simulink model "gm_UZ_EnDat_be4_segregation"  (R2023b)
settings: Solver=FixedStepAuto  StartTime=0  StopTime=0.000505  RelTol=1e-3
model workspace (MAT data in the model file):
  Select = 0
libraries: hdlsllib x74, simulink x21, hdlmdlgenlib x4, simulink_extras x1
(part 1 of 5)
settings Model: SimulationMode=accelerator  Creator=ELSYS_PC  LastModifiedBy=ELSYS_PC
settings SolverCC: AlgebraicLoopSolver=TrustRegion
settings DataIOCC: LimitDataPoints=on  SaveOutput=off  SaveTime=off
settings OptimizationCC: BlockReduction=off  ConditionallyExecuteInputs=off  DefaultParameterBehavior=Inlined  InheritOutputTypeSmallerThanSingle=on  LifeSpan=inf
settings DebuggingCC: AlgebraicLoopMsg=error  ArtificialAlgebraicLoopMsg=none  InheritedTsInSrcMsg=none  SingleTaskRateTransMsg=error  UnconnectedInputMsg=warning  UnconnectedOutputMsg=warning  UnconnectedLineMsg=warning  AllowSymbolicDim=off  StrictBusMsg=ErrorOnBusTreatedAsVector  SFUnexpectedBacktrackingDiag=warning  SFNoUnconditionalDefaultTransitionDiag=warning  SFExecutionAtInitializationDiag=none  ArithmeticOperatorsInVariantConditions=warning
settings HardwareCC: ProdBitPerPointer=32  ProdBitPerSizeT=32  ProdBitPerPtrDiffT=32  ProdLargestAtomicFloat=None  ProdIntDivRoundTo=Undefined  ProdEndianess=Unspecified  ProdWordSize=32  ProdHWDeviceType=ASIC/FPGA->ASIC/FPGA  ProdEqTarget=off
settings ModelReferenceCC: EnableRefExpFcnMdlSchedulingChecks=on
settings SFSimCC: SimUseLocalCustomCode=off  CustomCodeUndefinedFunction=UseInterfaceOnly
settings RTWCC: RTWUseLocalCustomCode=off
settings CodeAppCC: StateflowObjectComments=on
settings GRTTargetCC: TargetLangStandard=C89/C90 (ANSI)  RTWCAPISignals=on  RTWCAPIParams=on
settings ConfigComp: CovScope=ReferencedModels  CovMetricSettings=dw  CovSaveCumulativeToWorkspaceVar=on  CovSaveSingleToWorkspaceVar=on  CovExternalEMLEnable=off  CovSFcnEnable=off  DVTestSuiteOptimization=Auto  DVDetectOutOfBounds=on  DVModelReferenceHarness=on  DVHarnessSource=Signal Editor  DVRebuildModelRepresentation=IfChangeIsDetected

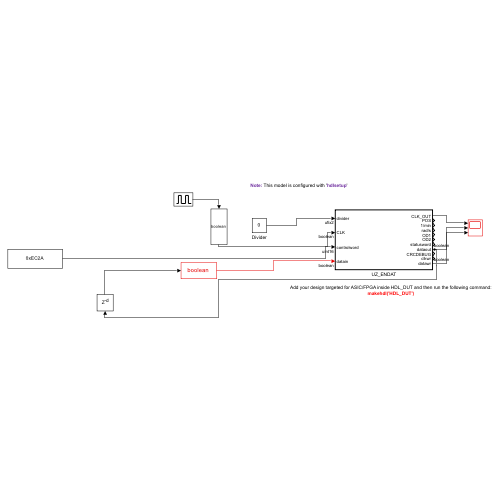
[thumbnail: Simulink's stored preview of the top-level diagram]
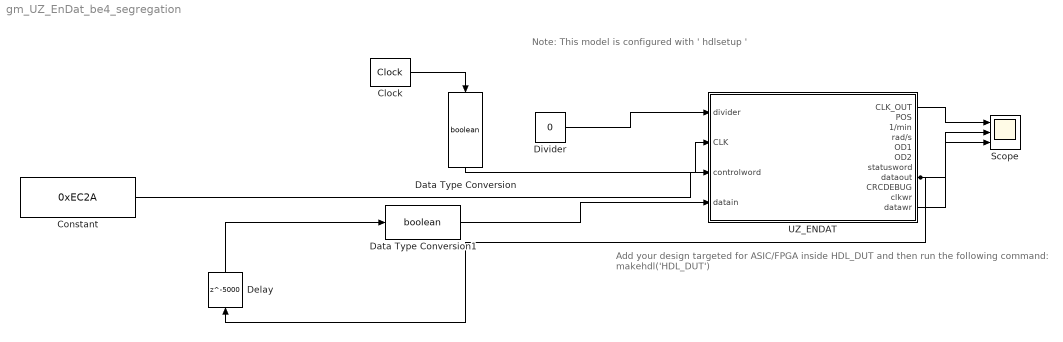
== system gm_UZ_EnDat_be4_segregation ==
  note: Add your design targeted for ASIC/FPGA inside HDL_DUT and then run the following command:
      | makehdl('HDL_DUT')
  note: Note: This model is configured with ' hdlsetup '
  Clock : simulink_extras/Flip Flops/Clock  period=2E-8
  Constant : Constant  Value=0xEC2A  OutDataTypeStr=uint16  SampleTime=-1
  Data Type Conversion : DataTypeConversion  OutDataTypeStr=boolean  SaturateOnIntegerOverflow=off  RndMeth=Floor
  Data Type Conversion1 : DataTypeConversion  OutDataTypeStr=boolean  SaturateOnIntegerOverflow=off  RndMeth=Floor
  Delay : Delay  DelayLength=5000
  Divider : Constant  Value=0  OutMin=0  OutMax=3  OutDataTypeStr=fixdt(0,2,0)  SampleTime=-1
  Scope : Scope  NumInputPorts=3
  UZ_ENDAT : Subsystem  TreatAsAtomicUnit=on
  wires:
  UZ_ENDAT/11(datawr) -> Scope/3
  UZ_ENDAT/1(CLK_OUT) -> Scope/1
  Delay/1 -> Data Type Conversion1/1
  UZ_ENDAT/8(dataout) -> Delay/1, Scope/2
  Data Type Conversion1/1 -> UZ_ENDAT/4(datain)
  Clock/1 -> Data Type Conversion/1
  Divider/1 -> UZ_ENDAT/1(divider)
  Data Type Conversion/1 -> UZ_ENDAT/2(CLK)
  Constant/1 -> UZ_ENDAT/3(controlword)

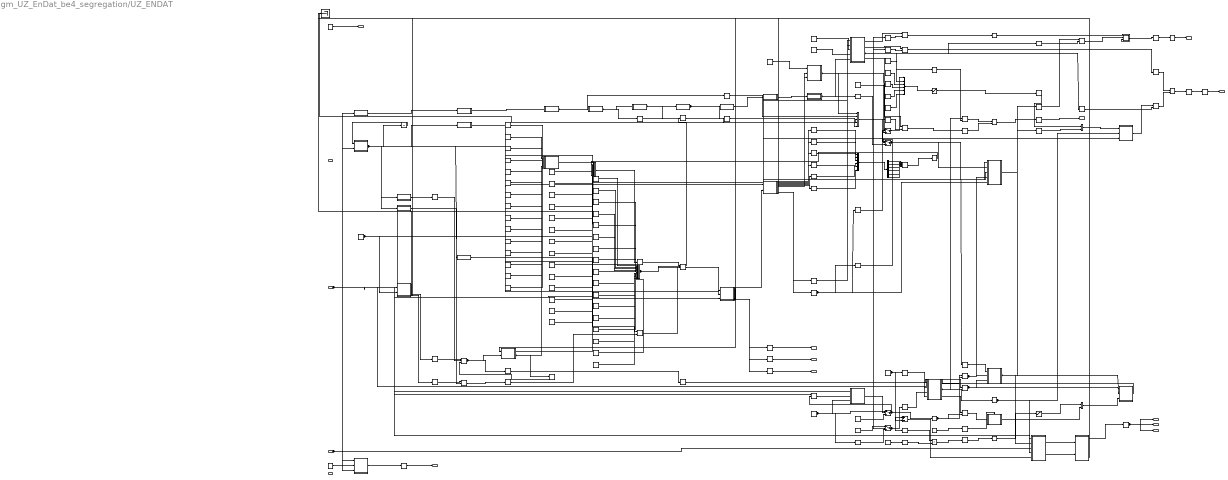
== system gm_UZ_EnDat_be4_segregation/UZ_ENDAT ==
  note: 0=12.5;1=6,25;2=3,125;3=1,5625
  divider : Inport  OutDataTypeStr=fixdt(0, 2, 0)  PortDimensions=1  SampleTime=1e-08
  CLK : Inport  Port=2  OutDataTypeStr=boolean  PortDimensions=1  SampleTime=1e-08
  controlword : Inport  Port=3  OutDataTypeStr=uint16  PortDimensions=1  SampleTime=1e-08
  datain : Inport  Port=4  OutDataTypeStr=boolean  PortDimensions=1  SampleTime=1e-08
  16BIT_SPLITTER : Subsystem
  16BIT_SPLITTER_term{2..14} (13 alike) : Terminator
  16bitgather : Subsystem
  2CLKDELAY : simulink/Discrete/Tapped Delay  vinit=0  samptime=-1  NumDelays=double(1024)  DelayOrder=Newest  includeCurrent=on
  5timestorage : Subsystem
  5timestorage_term{1..4} (4 alike) : Terminator
  CLKCNTER_ACT : Subsystem
  CLKCNTER_RAMPUP : Subsystem
  CLKDIV1 : Subsystem
  CLKDIV2 : Subsystem
  CLKDIV3 : Subsystem
  CLKDIV4 : Subsystem
  CLKDIV5 : Subsystem
  CLKDIV6 : Subsystem
  CLKDIV7 : Subsystem
  CLKDIV8 : Subsystem
  CLKDIV9 : Subsystem
  CONTROLWORDRAW : Subsystem
  CONTROLWORDRAW_term{0..12,14} (14 alike) : Terminator
  CONTROLWORDSTORED : Subsystem
  CONTROLWORDSTORED_term{7..13,15} (8 alike) : Terminator
  CRC_Check : Subsystem
  Compare To Constant : Subsystem  mask(Compare To Constant){relop===, const=double(1), OutDataTypeStr=boolean, ZeroCross=on}
      mask prompts: relop "Simulink:masks:Operator_MP"; const "Simulink:masks:ConstantValue_MP"; OutDataTypeStr "Simulink:masks:OutputDataType_MP"; ZeroCross "Simulink:masks:EnableZerocrossingDetection_MP"
      mask help: Simulink:masks:CompareToConstant_MD
      mask init:
      | OutDataTypeStr = 'boolean';
      | ZeroCross = 'on';
      | blkName = 'UZ_EnDat_be4_segregation/UZ_ENDAT/Compare\nTo Constant';
      | const = double(1);
      | const_str = '1';
      | const_val = double(1);
      | relop = '==';
      | setValue = 'boolean';
      | str = '== 1';
      mask TypeOptions relop: == | ~= | < | <= | >= | >
      mask TypeOptions OutDataTypeStr: Simulink:masks:uint8 | Simulink:masks:boolean
      mask Callback ZeroCross: sl('zeroCrossEnable', gcbh);
      mask Display: disp(str)
  Compare To Constant1 : Subsystem  mask(Compare To Constant){relop===, const=double(1), OutDataTypeStr=boolean, ZeroCross=on}
      mask prompts: relop "Simulink:masks:Operator_MP"; const "Simulink:masks:ConstantValue_MP"; OutDataTypeStr "Simulink:masks:OutputDataType_MP"; ZeroCross "Simulink:masks:EnableZerocrossingDetection_MP"
      mask help: Simulink:masks:CompareToConstant_MD
      mask init:
      | OutDataTypeStr = 'boolean';
      | ZeroCross = 'on';
      | blkName = 'UZ_EnDat_be4_segregation/UZ_ENDAT/Compare\nTo Constant1';
      | const = double(1);
      | const_str = '1';
      | const_val = double(1);
      | relop = '==';
      | setValue = 'boolean';
      | str = '== 1';
      mask TypeOptions relop: == | ~= | < | <= | >= | >
      mask TypeOptions OutDataTypeStr: Simulink:masks:uint8 | Simulink:masks:boolean
      mask Callback ZeroCross: sl('zeroCrossEnable', gcbh);
      mask Display: disp(str)
  Compare To Constant2 : Subsystem  mask(Compare To Constant){relop===, const=double(0), OutDataTypeStr=boolean, ZeroCross=on}
      mask prompts: relop "Simulink:masks:Operator_MP"; const "Simulink:masks:ConstantValue_MP"; OutDataTypeStr "Simulink:masks:OutputDataType_MP"; ZeroCross "Simulink:masks:EnableZerocrossingDetection_MP"
      mask help: Simulink:masks:CompareToConstant_MD
      mask init:
      | OutDataTypeStr = 'boolean';
      | ZeroCross = 'on';
      | blkName = 'UZ_EnDat_be4_segregation/UZ_ENDAT/Compare\nTo Constant2';
      | const = double(0);
      | const_str = '0';
      | const_val = double(0);
      | relop = '==';
      | setValue = 'boolean';
      | str = '== 0';
      mask TypeOptions relop: == | ~= | < | <= | >= | >
      mask TypeOptions OutDataTypeStr: Simulink:masks:uint8 | Simulink:masks:boolean
      mask Callback ZeroCross: sl('zeroCrossEnable', gcbh);
      mask Display: disp(str)
  Constant : Constant  OutDataTypeStr=boolean  SampleTime=1e-08
  Constant1 : Constant  Value=1023  OutDataTypeStr=uint16  SampleTime=1e-08
  Constant10 : Constant  Value=3  OutDataTypeStr=fixdt(0, 2, 0)  SampleTime=1e-08
  Constant11 : Constant  Value=44039  OutDataTypeStr=uint16  SampleTime=1e-08
  Constant12 : Constant  Value=48  OutDataTypeStr=uint16  SampleTime=1e-08
  Constant13 : Constant  Value=8  OutDataTypeStr=uint8  SampleTime=1e-08
  Constant2 : Constant  Value=16  OutDataTypeStr=uint16  SampleTime=1e-08
  Constant3 : Constant  OutDataTypeStr=boolean  SampleTime=1e-08
  Constant4 : Constant  Value=32  OutDataTypeStr=uint16  SampleTime=1e-08
  Constant5 : Constant  Value=0  OutDataTypeStr=uint8  SampleTime=1e-08
  Constant6 : Constant  Value=300  OutDataTypeStr=uint16  SampleTime=1e-08
  Constant7 : Constant  Value=64  OutDataTypeStr=uint16  SampleTime=1e-08
  Constant8 : Constant  Value=128  OutDataTypeStr=uint16  SampleTime=1e-08
  Constant9 : Constant  Value=4  OutDataTypeStr=uint8  SampleTime=1e-08
  ControlWordRAM : Constant  Value=0  VectorParams1D=off  OutDataTypeStr=uint8  SampleTime=1e-08
  Data Type Conversion1 : Subsystem
      mask Display: disp('NFP\nconv');
  Data Type Conversion10 : DataTypeConversion  OutDataTypeStr=uint16  RndMeth=Nearest  SampleTime=1e-08  SaturateOnIntegerOverflow=off
  Data Type Conversion{4..9} (6 alike) : DataTypeConversion  OutDataTypeStr=fixdt(0, 1, 0)  SampleTime=1e-08  SaturateOnIntegerOverflow=off  RndMeth=Floor
  Delay : Delay  DelayLength=double(10)  InitialCondition=0  SampleTime=1e-08
  Delay1 : hdlmdlgenlib/Buffer
  Delay2 : Delay  DelayLength=double(1)  InitialCondition=0  SampleTime=1e-08
  Delay3 : Delay  DelayLength=double(1)  InitialCondition=0  SampleTime=1e-08
  Delay4 : hdlmdlgenlib/Buffer
  Delay5 : hdlmdlgenlib/Buffer
  Detect Change : simulink/Logic and Bit Operations/Detect Change  vinit=0  OutDataTypeStr=boolean
      settings: LibrarySourceBlock=|
      | hdlsllib/Logic and Bit
      | Operations/Detect
      | Change
  Dual Port RAM System : hdlsllib/HDL RAMs/Dual Port RAM System  RAMType=Dual port  AsyncRead=off  WriteOutputValue=New data  RAMInitialValue=0  allowBusInputs=off  WritesHaveOutput=on  NumReads=0  NumWrites=1  SimulateUsing=Code generation
  Dual Port RAM System_term0 : Terminator
  EndatControlRAM : Constant  VectorParams1D=off  OutDataTypeStr=uint8  SampleTime=1e-08
  Gain : Product  Inputs=**  OutDataTypeStr=fixdt(0, 32, 10)  SampleTime=1e-08
  Gain_const : Constant  Value=40  OutDataTypeStr=fixdt(0, 16, 10)  SampleTime=1e-08
  Gain_out_dtc : DataTypeConversion  OutDataTypeStr=uint16  SampleTime=1e-08  RndMeth=Floor
  HwModeRegister : Delay  DelayLength=double(1)  InitialCondition=0  SampleTime=1e-08
  HwModeRegister1 : Delay  DelayLength=double(1)  InitialCondition=0  SampleTime=1e-08
  Logical Operator{,1,7,9,13..14,16,18,20} (9 alike) : Logic  AllPortsSameDT=off  OutDataTypeStr=boolean  SampleTime=1e-08
  Logical Operator{2..4,6,10,12,17,19,21,24} (10 alike) : Logic  Operator=NOT  Inputs=1  AllPortsSameDT=off  OutDataTypeStr=boolean  SampleTime=1e-08
  Logical Operator{5,11,15,22..23} (5 alike) : Logic  Operator=OR  AllPortsSameDT=off  OutDataTypeStr=boolean  SampleTime=1e-08
  Logical Operator8 : Logic  Inputs=3  AllPortsSameDT=off  OutDataTypeStr=boolean  SampleTime=1e-08
  ManualDeserializere : Subsystem
  ManualSerialize : Subsystem
  Memory : UnitDelay  InitialCondition="fi(0,0,4,0,\"hex\",\"0\")"  SampleTime=1e-08
  Multiport Switch : MultiPortSwitch  DataPortOrder=Zero-based contiguous  Inputs=4  DiagnosticForDefault=None  zeroidx=on  SampleTime=1e-08  SaturateOnIntegerOverflow=off  InputSameDT=off
  Multiport Switch1 : MultiPortSwitch  DataPortOrder=Zero-based contiguous  Inputs=5  DiagnosticForDefault=None  zeroidx=on  OutDataTypeStr=uint16  SampleTime=1e-08  SaturateOnIntegerOverflow=off  InputSameDT=off
  OUTPUTCONTROLCONTINIOUS : Subsystem
  PipelineRegister : Delay  DelayLength=double(1)  InitialCondition=0  SampleTime=1e-08
  RAM_SELECTOR : MultiPortSwitch  DataPortOrder=Zero-based contiguous  Inputs=16  DataPortForDefault=Additional data port  DiagnosticForDefault=None  zeroidx=on  OutDataTypeStr=uint8  SampleTime=1e-08  SaturateOnIntegerOverflow=off  InputSameDT=off
  RAM_SELECTOR1 : MultiPortSwitch  DataPortOrder=Zero-based contiguous  Inputs=16  DataPortForDefault=Additional data port  DiagnosticForDefault=None  zeroidx=on  OutDataTypeStr=uint16  SampleTime=1e-08  SaturateOnIntegerOverflow=off  InputSameDT=off
  RECOVERYTIME : Subsystem
      settings: MinAlgLoopOccurrences=on
  SetZero : Subsystem
  SetZeroBool : Subsystem
  SetZeroBool1 : Subsystem
  Signal Specification : SignalSpecification  OutDataTypeStr=uint16  Dimensions=1
  StatusWordRAM : Constant  Value=15  VectorParams1D=off  OutDataTypeStr=uint8  SampleTime=1e-08
  Storage16 : Subsystem
  Subsystem : Subsystem
  Subtract : Sum  Inputs=+-  OutDataTypeStr=uint16  AccumDataTypeStr=uint16  SampleTime=1e-08
  Switch : Switch  Criteria=u2 ~= 0  Threshold=double(0)  OutDataTypeStr=boolean  SampleTime=1e-08  SaturateOnIntegerOverflow=off  InputSameDT=off
  Switch1 : Switch  Criteria=u2 ~= 0  Threshold=double(0)  OutDataTypeStr=uint8  SampleTime=1e-08  SaturateOnIntegerOverflow=off  InputSameDT=off
  TmpGroundAt16bitgatherInport{1..13,15..16} (15 alike) : Constant  Value=0  VectorParams1D=off  OutDataTypeStr=boolean  SampleTime=1e-08
  TmpGroundAtRAM_SELECTOR1Inport{4..16,18} (14 alike) : Constant  Value=0  VectorParams1D=off  OutDataTypeStr=uint16  SampleTime=1e-08
  TmpGroundAtRAM_SELECTORInport{4..16,18} (14 alike) : Constant  Value=0  VectorParams1D=off  OutDataTypeStr=uint8  SampleTime=1e-08
  concat : hdlsllib/Logic and Bit Operations/Bit Concat  numInputs=6
  concatenate : Concatenate  NumInputs=6
  deadtime : Switch  Threshold=double(2000)  OutDataTypeStr=boolean  SampleTime=1e-08  SaturateOnIntegerOverflow=off  InputSameDT=off
  deadtime1 : Switch  Criteria=u2 ~= 0  Threshold=double(0)  OutDataTypeStr=uint16  SampleTime=1e-08  SaturateOnIntegerOverflow=off  InputSameDT=off
  deadtimeconst1 : Constant  OutDataTypeStr=boolean  SampleTime=1e-08
  deadtimeconst2 : Constant  Value=0  OutDataTypeStr=boolean  SampleTime=1e-08
  delayMatch{,1..5,12,15..16} (9 alike) : Delay  DelayLength=double(1)  InitialCondition=0  SampleTime=1e-08
  delayMatch{6..11,13..14,17..20} (12 alike) : Delay  DelayLength=double(2)  InitialCondition=0  SampleTime=1e-08
  delayMatch21 : Delay  DelayLength=double(3)  InitialCondition=0  SampleTime=1e-08
  delayMatch{22..24,26} (4 alike) : Delay  DelayLength=double(5)  InitialCondition=0  SampleTime=1e-08
  delayMatch25 : Delay  DelayLength=double(3)  InitialCondition=0  SampleTime=1e-08
  delayMatch27 : Delay  DelayLength=double(3)  InitialCondition=0  SampleTime=1e-08
  multiportswitch : MultiPortSwitch  DataPortOrder=Zero-based contiguous  Inputs=1  DiagnosticForDefault=None  zeroidx=on  SampleTime=1e-08  SaturateOnIntegerOverflow=off  InputSameDT=off
  multiportswitch1 : MultiPortSwitch  DataPortOrder=Zero-based contiguous  Inputs=1  DiagnosticForDefault=None  zeroidx=on  SampleTime=1e-08  SaturateOnIntegerOverflow=off  InputSameDT=off
  ramselektor : Subsystem
  saturate : Saturate  UpperLimit=double(1024)  LowerLimit=double(0)  SampleTime=1e-08  OutDataTypeStr=uint16
  saturate1 : Saturate  UpperLimit=double(2000)  LowerLimit=double(0)  SampleTime=1e-08  OutDataTypeStr=uint16
  stateControl : Constant  OutDataTypeStr=boolean  SampleTime=1e-08
  t : Demux  Outputs=6
  CLK_OUT : Outport  SampleTime=1e-08  VectorParamsAs1DForOutWhenUnconnected=off
  POS : Outport  Port=2  OutDataTypeStr=double  SampleTime=1e-08  VectorParamsAs1DForOutWhenUnconnected=off
  1/min : Outport  Port=3  OutDataTypeStr=double  SampleTime=1e-08  VectorParamsAs1DForOutWhenUnconnected=off
  rad/s : Outport  Port=4  OutDataTypeStr=double  SampleTime=1e-08  VectorParamsAs1DForOutWhenUnconnected=off
  OD1 : Outport  Port=5  OutDataTypeStr=uint16  SampleTime=1e-08  VectorParamsAs1DForOutWhenUnconnected=off
  OD2 : Outport  Port=6  OutDataTypeStr=uint16  SampleTime=1e-08  VectorParamsAs1DForOutWhenUnconnected=off
  statusword : Outport  Port=7  OutDataTypeStr=uint16  SampleTime=1e-08  VectorParamsAs1DForOutWhenUnconnected=off
  dataout : Outport  Port=8  OutDataTypeStr=boolean  SampleTime=1e-08  VectorParamsAs1DForOutWhenUnconnected=off
  CRCDEBUG : Outport  Port=9  OutDataTypeStr=boolean  SampleTime=1e-08  VectorParamsAs1DForOutWhenUnconnected=off
  clkwr : Outport  Port=10  OutDataTypeStr=boolean  SampleTime=1e-08  VectorParamsAs1DForOutWhenUnconnected=off
  datawr : Outport  Port=11  OutDataTypeStr=boolean  SampleTime=1e-08  VectorParamsAs1DForOutWhenUnconnected=off
  wires:
  datain/1 -> ManualSerialize/3(DATA), CRC_Check/1(data)
  delayMatch22/1 -> OD1/1
  multiportswitch/1 -> SetZeroBool1/1(valin)
  5timestorage/1(t0) -> Data Type Conversion1/1(In1)
  CLKDIV1/1(CLK/2) -> CLKDIV3/1(CLK1)
  CLKDIV2/1(CLK/2) -> CLKDIV1/1(CLK1)
  delayMatch/1 -> Multiport Switch/2
  delayMatch1/1 -> Multiport Switch/3
  delayMatch2/1 -> Multiport Switch/4
  delayMatch3/1 -> Multiport Switch/5
  CLKDIV7/1(CLK/2) -> CLKDIV8/1(CLK1)
  CLKDIV8/1(CLK/2) -> CLKDIV9/1(CLK1)
  delayMatch5/1 -> Switch/3
  CONTROLWORDRAW/14(DATAOUT13) -> Delay2/1
  CONTROLWORDRAW/16(DATAOUT15) -> Logical Operator3/1
  CONTROLWORDSTORED/7(DATAOUT6) -> SetZero/2(setzero)
  CONTROLWORDSTORED/15(DATAOUT14) -> Logical Operator24/1, Logical Operator12/1
  delayMatch26/1 -> CRCDEBUG/1
  Compare To Constant/1(y) -> Logical Operator1/2
  Compare To Constant1/1(y) -> Delay3/1
  Constant/1 -> CRC_Check/2(set)
  Constant1/1 -> Multiport Switch1/6
  Constant10/1 -> SetZero/1(valin)
  Constant11/1 -> CONTROLWORDRAW/2(DATA), RAM_SELECTOR1/2
  Constant12/1 -> Subsystem/4(CLK2ENDOFTRANSMISSION)
  Constant13/1 -> Subsystem/3(CLKS2DATAFLOWCHG)
  Constant2/1 -> Multiport Switch1/2
  Constant3/1 -> clkwr/1
  Constant4/1 -> Multiport Switch1/3
  Constant6/1 -> deadtime1/1
  Constant7/1 -> Multiport Switch1/4
  Constant8/1 -> Multiport Switch1/5
  Constant9/1 -> Switch1/3
  ControlWordRAM/1 -> RAM_SELECTOR/2
  Data Type Conversion10/1 -> deadtime1/3
  delayMatch25/1 -> dataout/1
  Delay4/1 -> Logical Operator13/1
  delayMatch21/1 -> CLK_OUT/1
  Detect Change/1 -> Logical Operator/1
  Dual Port RAM System/1 -> Dual Port RAM System_term0/1
  EndatControlRAM/1 -> RAM_SELECTOR/3
  Gain_out_dtc/1 -> saturate1/1
  Logical Operator1/1 -> Logical Operator2/1
  delayMatch4/1 -> Switch/2
  Logical Operator13/1 -> Logical Operator22/1
  Logical Operator14/1 -> Logical Operator15/1
  delayMatch27/1 -> datawr/1
  delayMatch20/1 -> Logical Operator15/2
  Logical Operator17/1 -> Logical Operator16/2
  delayMatch14/1 -> Logical Operator22/2
  Logical Operator19/1 -> Logical Operator18/2
  Logical Operator2/1 -> Logical Operator/2
  delayMatch18/1 -> Logical Operator23/1
  Logical Operator21/1 -> Logical Operator20/2
  Logical Operator22/1 -> Delay5/1
  Logical Operator23/1 -> Delay1/1
  Logical Operator24/1 -> Subsystem/2(RESET)
  Logical Operator3/1 -> Logical Operator1/1
  Logical Operator4/1 -> ManualSerialize/4(recieving), SetZeroBool1/2(setzero)
  Logical Operator8/1 -> Logical Operator10/1, Storage16/2(Write)
  Logical Operator9/1 -> Logical Operator23/2
  ManualDeserializere/1(valin) -> 2CLKDELAY/1
  ManualSerialize/1(valueout) -> 5timestorage/1(DATA)
  ManualSerialize/2(wrok) -> 5timestorage/2(wrok)
  Multiport Switch/1 -> Switch/1
  Multiport Switch1/1 -> saturate/1
  SetZero/1(valueout) -> Switch1/1, Multiport Switch/1
  SetZeroBool1/1(valueout) -> Logical Operator9/1
  StatusWordRAM/1 -> RAM_SELECTOR/17
  Storage16/1(out) -> ManualDeserializere/3(DATA)
  Subsystem/1(CLKOUT) -> Logical Operator18/1
  Subsystem/2(DATAOUT) -> Logical Operator20/1
  delayMatch13/1 -> Logical Operator13/2
  Subsystem/4(DATAINV) -> Logical Operator16/1
  Subtract/1 -> ManualSerialize/5(recievecnt)
  Switch1/1 -> Multiport Switch1/1
  TmpGroundAtRAM_SELECTORInport10/1 -> RAM_SELECTOR/10
  TmpGroundAtRAM_SELECTORInport11/1 -> RAM_SELECTOR/11
  TmpGroundAtRAM_SELECTORInport12/1 -> RAM_SELECTOR/12
  TmpGroundAtRAM_SELECTORInport13/1 -> RAM_SELECTOR/13
  TmpGroundAtRAM_SELECTORInport14/1 -> RAM_SELECTOR/14
  TmpGroundAtRAM_SELECTORInport15/1 -> RAM_SELECTOR/15
  TmpGroundAtRAM_SELECTORInport16/1 -> RAM_SELECTOR/16
  TmpGroundAtRAM_SELECTORInport18/1 -> RAM_SELECTOR/18
  TmpGroundAtRAM_SELECTORInport4/1 -> RAM_SELECTOR/4
  TmpGroundAtRAM_SELECTORInport5/1 -> RAM_SELECTOR/5
  TmpGroundAtRAM_SELECTORInport6/1 -> RAM_SELECTOR/6
  TmpGroundAtRAM_SELECTORInport7/1 -> RAM_SELECTOR/7
  TmpGroundAtRAM_SELECTORInport8/1 -> RAM_SELECTOR/8
  TmpGroundAtRAM_SELECTORInport9/1 -> RAM_SELECTOR/9
  deadtimeconst2/1 -> Data Type Conversion10/1, CLKCNTER_RAMPUP/3(ResetCNT), deadtime/1
  ramselektor/1(SEL) -> RAM_SELECTOR/1, Compare To Constant/1(u), Detect Change/1, Compare To Constant2/1(u), Compare To Constant1/1(u), Memory/1, 16BIT_SPLITTER/2(SEL), RAM_SELECTOR1/1
  2CLKDELAY/1 -> multiportswitch/2
  delayMatch16/1 -> multiportswitch/1
  16BIT_SPLITTER/3(DATAOUT2) -> 16BIT_SPLITTER_term2/1
  16BIT_SPLITTER/4(DATAOUT3) -> 16BIT_SPLITTER_term3/1
  16BIT_SPLITTER/5(DATAOUT4) -> 16BIT_SPLITTER_term4/1
  16BIT_SPLITTER/6(DATAOUT5) -> 16BIT_SPLITTER_term5/1
  16BIT_SPLITTER/7(DATAOUT6) -> 16BIT_SPLITTER_term6/1
  16BIT_SPLITTER/8(DATAOUT7) -> 16BIT_SPLITTER_term7/1
  16BIT_SPLITTER/9(DATAOUT8) -> 16BIT_SPLITTER_term8/1
  16BIT_SPLITTER/10(DATAOUT9) -> 16BIT_SPLITTER_term9/1
  16BIT_SPLITTER/11(DATAOUT10) -> 16BIT_SPLITTER_term10/1
  16BIT_SPLITTER/12(DATAOUT11) -> 16BIT_SPLITTER_term11/1
  16BIT_SPLITTER/13(DATAOUT12) -> 16BIT_SPLITTER_term12/1
  16BIT_SPLITTER/14(DATAOUT13) -> 16BIT_SPLITTER_term13/1
  16BIT_SPLITTER/15(DATAOUT14) -> 16BIT_SPLITTER_term14/1
  5timestorage/2(t-1) -> 5timestorage_term1/1
  5timestorage/3(t-2) -> 5timestorage_term2/1
  5timestorage/4(t-3) -> 5timestorage_term3/1
  5timestorage/5(t-4) -> 5timestorage_term4/1
  CONTROLWORDRAW/1(DATAOUT0) -> CONTROLWORDRAW_term0/1
  CONTROLWORDRAW/2(DATAOUT1) -> CONTROLWORDRAW_term1/1
  CONTROLWORDRAW/3(DATAOUT2) -> CONTROLWORDRAW_term2/1
  CONTROLWORDRAW/4(DATAOUT3) -> CONTROLWORDRAW_term3/1
  CONTROLWORDRAW/5(DATAOUT4) -> CONTROLWORDRAW_term4/1
  CONTROLWORDRAW/6(DATAOUT5) -> CONTROLWORDRAW_term5/1
  CONTROLWORDRAW/7(DATAOUT6) -> CONTROLWORDRAW_term6/1
  CONTROLWORDRAW/8(DATAOUT7) -> CONTROLWORDRAW_term7/1
  CONTROLWORDRAW/9(DATAOUT8) -> CONTROLWORDRAW_term8/1
  CONTROLWORDRAW/10(DATAOUT9) -> CONTROLWORDRAW_term9/1
  CONTROLWORDRAW/11(DATAOUT10) -> CONTROLWORDRAW_term10/1
  CONTROLWORDRAW/12(DATAOUT11) -> CONTROLWORDRAW_term11/1
  CONTROLWORDRAW/13(DATAOUT12) -> CONTROLWORDRAW_term12/1
  CONTROLWORDRAW/15(DATAOUT14) -> CONTROLWORDRAW_term14/1
  CONTROLWORDSTORED/8(DATAOUT7) -> CONTROLWORDSTORED_term7/1
  CONTROLWORDSTORED/9(DATAOUT8) -> CONTROLWORDSTORED_term8/1
  CONTROLWORDSTORED/10(DATAOUT9) -> CONTROLWORDSTORED_term9/1
  CONTROLWORDSTORED/11(DATAOUT10) -> CONTROLWORDSTORED_term10/1
  CONTROLWORDSTORED/12(DATAOUT11) -> CONTROLWORDSTORED_term11/1
  CONTROLWORDSTORED/13(DATAOUT12) -> CONTROLWORDSTORED_term12/1
  CONTROLWORDSTORED/14(DATAOUT13) -> CONTROLWORDSTORED_term13/1
  CONTROLWORDSTORED/16(DATAOUT15) -> CONTROLWORDSTORED_term15/1
  Gain_const/1 -> HwModeRegister1/1
  PipelineRegister/1 -> Gain_out_dtc/1
  Data Type Conversion1/1(Out1) -> POS/1, rad/s/1, 1/min/1
  CLKDIV3/1(CLK/2) -> delayMatch/1, CLKDIV4/1(CLK1)
  CLKDIV4/1(CLK/2) -> delayMatch1/1, CLKDIV5/1(CLK1)
  CLKDIV5/1(CLK/2) -> delayMatch2/1, CLKDIV6/1(CLK1)
  CLKDIV6/1(CLK/2) -> delayMatch3/1, CLKDIV7/1(CLK1)
  delayMatch15/1 -> Switch1/2
  CLKDIV9/1(CLK/2) -> delayMatch5/1, Subsystem/5(VERYSLOWCLK)
  deadtime/1 -> delayMatch6/1, Logical Operator7/2
  stateControl/1 -> delayMatch7/1
  CLK/1 -> delayMatch8/1, ManualSerialize/1(CLK), CRC_Check/3(clk), SetZeroBool1/3(Trigger), ManualDeserializere/1(CLK), Subsystem/1(CLK), SetZero/3(Trigger), CONTROLWORDRAW/1(CLK), CLKDIV2/1(CLK1), CLKCNTER_RAMPUP/1(CLK), Logical Operator7/1, ramselektor/2(Trigger), 16BIT_SPLITTER/3(Trigger)
  Constant5/1 -> delayMatch9/1, Subtract/2
  deadtime1/1 -> delayMatch10/1, Subtract/1, HwModeRegister/1
  Logical Operator10/1 -> delayMatch11/1
  Switch/1 -> delayMatch12/1, ManualDeserializere/2(SLOWCLCK)
  delayMatch17/1 -> Logical Operator9/2
  Logical Operator18/1 -> delayMatch14/1
  Logical Operator12/1 -> delayMatch15/1, delayMatch4/1, ManualDeserializere/5(14)
  saturate/1 -> delayMatch16/1
  delayMatch19/1 -> Logical Operator14/2
  Logical Operator20/1 -> delayMatch18/1
  Subsystem/3(BOOTUPCOMPLETE) -> delayMatch19/1, delayMatch17/1, delayMatch13/1, deadtime1/2, Logical Operator21/1, Logical Operator19/1, Logical Operator17/1
  Logical Operator16/1 -> delayMatch20/1
  Delay5/1 -> delayMatch21/1
  delayMatch23/1 -> OD2/1
  delayMatch24/1 -> statusword/1
  16BIT_SPLITTER/16(DATAOUT15) -> delayMatch24/1, delayMatch23/1, delayMatch22/1
  Delay1/1 -> delayMatch25/1
  CRC_Check/1(crc) -> delayMatch26/1
  Logical Operator15/1 -> delayMatch27/1
  OUTPUTCONTROLCONTINIOUS/2(DATAINV) -> Logical Operator4/1, Logical Operator14/1
  Logical Operator11/1 -> SetZeroBool/2(setzero), ManualDeserializere/4(reset)
  SetZeroBool/1(valueout) -> CLKCNTER_ACT/2(CLK2CNT), Delay4/1, ManualSerialize/2(SLOWCLCK)
  multiportswitch1/1 -> CLKCNTER_ACT/3(ResetCNT)
  delayMatch8/1 -> CLKCNTER_ACT/1(CLK), SetZeroBool/3(Trigger)
  delayMatch12/1 -> SetZeroBool/1(valin)
  delayMatch6/1 -> Logical Operator11/2, Logical Operator5/2
  delayMatch7/1 -> RECOVERYTIME/Enable
  saturate1/1 -> multiportswitch1/1
  CLKCNTER_ACT/1(CNT) -> OUTPUTCONTROLCONTINIOUS/1(CLKCNT)
  delayMatch9/1 -> OUTPUTCONTROLCONTINIOUS/2(CLKS2DATAFLOWCHG)
  delayMatch10/1 -> OUTPUTCONTROLCONTINIOUS/3(CLK2ENDOFTRANSMISSION)
  delayMatch11/1 -> OUTPUTCONTROLCONTINIOUS/4(OPENCOM)
  OUTPUTCONTROLCONTINIOUS/1(CLKOFF) -> Logical Operator11/1
  OUTPUTCONTROLCONTINIOUS/3(RESETCNT) -> Logical Operator5/1
  Memory/1 -> ramselektor/1(In1)
  Compare To Constant2/1(y) -> CONTROLWORDSTORED/1(CLK)
  16BIT_SPLITTER/1(DATAOUT0) -> CONTROLWORDSTORED/2(DATA)
  Dual Port RAM System/2 -> 16BIT_SPLITTER/1(DATAIN)
  TmpGroundAt16bitgatherInport1/1 -> 16bitgather/1(1)
  TmpGroundAt16bitgatherInport2/1 -> 16bitgather/2(In2)
  TmpGroundAt16bitgatherInport3/1 -> 16bitgather/3(In3)
  TmpGroundAt16bitgatherInport4/1 -> 16bitgather/4(In4)
  TmpGroundAt16bitgatherInport5/1 -> 16bitgather/5(In5)
  TmpGroundAt16bitgatherInport6/1 -> 16bitgather/6(In6)
  TmpGroundAt16bitgatherInport7/1 -> 16bitgather/7(In7)
  TmpGroundAt16bitgatherInport8/1 -> 16bitgather/8(In8)
  TmpGroundAt16bitgatherInport9/1 -> 16bitgather/9(In9)
  TmpGroundAt16bitgatherInport10/1 -> 16bitgather/10(In10)
  TmpGroundAt16bitgatherInport11/1 -> 16bitgather/11(In11)
  TmpGroundAt16bitgatherInport12/1 -> 16bitgather/12(In12)
  TmpGroundAt16bitgatherInport13/1 -> 16bitgather/13(In13)
  TmpGroundAt16bitgatherInport15/1 -> 16bitgather/15(In15)
  TmpGroundAt16bitgatherInport16/1 -> 16bitgather/16(In1)
  Delay/1 -> RAM_SELECTOR1/3
  TmpGroundAtRAM_SELECTOR1Inport4/1 -> RAM_SELECTOR1/4
  TmpGroundAtRAM_SELECTOR1Inport5/1 -> RAM_SELECTOR1/5
  TmpGroundAtRAM_SELECTOR1Inport6/1 -> RAM_SELECTOR1/6
  TmpGroundAtRAM_SELECTOR1Inport7/1 -> RAM_SELECTOR1/7
  TmpGroundAtRAM_SELECTOR1Inport8/1 -> RAM_SELECTOR1/8
  TmpGroundAtRAM_SELECTOR1Inport9/1 -> RAM_SELECTOR1/9
  TmpGroundAtRAM_SELECTOR1Inport10/1 -> RAM_SELECTOR1/10
  TmpGroundAtRAM_SELECTOR1Inport11/1 -> RAM_SELECTOR1/11
  TmpGroundAtRAM_SELECTOR1Inport12/1 -> RAM_SELECTOR1/12
  TmpGroundAtRAM_SELECTOR1Inport13/1 -> RAM_SELECTOR1/13
  TmpGroundAtRAM_SELECTOR1Inport14/1 -> RAM_SELECTOR1/14
  TmpGroundAtRAM_SELECTOR1Inport15/1 -> RAM_SELECTOR1/15
  TmpGroundAtRAM_SELECTOR1Inport16/1 -> RAM_SELECTOR1/16
  TmpGroundAtRAM_SELECTOR1Inport18/1 -> RAM_SELECTOR1/18
  RAM_SELECTOR/1 -> Dual Port RAM System/2, Dual Port RAM System/4
  Logical Operator/1 -> Dual Port RAM System/3
  16BIT_SPLITTER/2(DATAOUT1) -> Storage16/1(Data)
  Delay2/1 -> Logical Operator8/1
  Delay3/1 -> Logical Operator8/2
  16bitgather/1(Out1) -> RAM_SELECTOR1/17
  RAM_SELECTOR1/1 -> Signal Specification/1
  Signal Specification/1 -> Dual Port RAM System/1
  Storage16/2(wrok) -> 16bitgather/14(wrok), Logical Operator6/1
  Logical Operator6/1 -> Logical Operator8/3
  concat/1 -> Delay/1
  CONTROLWORDSTORED/6(DATAOUT5) -> Data Type Conversion9/1
  CONTROLWORDSTORED/5(DATAOUT4) -> Data Type Conversion8/1
  CONTROLWORDSTORED/4(DATAOUT3) -> Data Type Conversion7/1
  CONTROLWORDSTORED/3(DATAOUT2) -> Data Type Conversion6/1
  CONTROLWORDSTORED/2(DATAOUT1) -> Data Type Conversion5/1
  CONTROLWORDSTORED/1(DATAOUT0) -> Data Type Conversion4/1
  Data Type Conversion9/1 -> concatenate/6
  Data Type Conversion8/1 -> concatenate/5
  Data Type Conversion7/1 -> concatenate/4
  Data Type Conversion6/1 -> concatenate/3
  Data Type Conversion5/1 -> concatenate/2
  Data Type Conversion4/1 -> concatenate/1
  concatenate/1 -> t/1
  t/1 -> concat/6
  t/2 -> concat/5
  t/3 -> concat/4
  t/4 -> concat/3
  t/5 -> concat/2
  t/6 -> concat/1
  Logical Operator7/1 -> CLKCNTER_RAMPUP/2(CLK2CNT)
  CLKCNTER_RAMPUP/1(CNT) -> deadtime/2
  deadtimeconst1/1 -> deadtime/3
  RECOVERYTIME/1(out0) -> multiportswitch1/2
  Logical Operator5/1 -> RECOVERYTIME/1(in0)
  Gain/1 -> PipelineRegister/1
  HwModeRegister/1 -> Gain/1
  HwModeRegister1/1 -> Gain/2

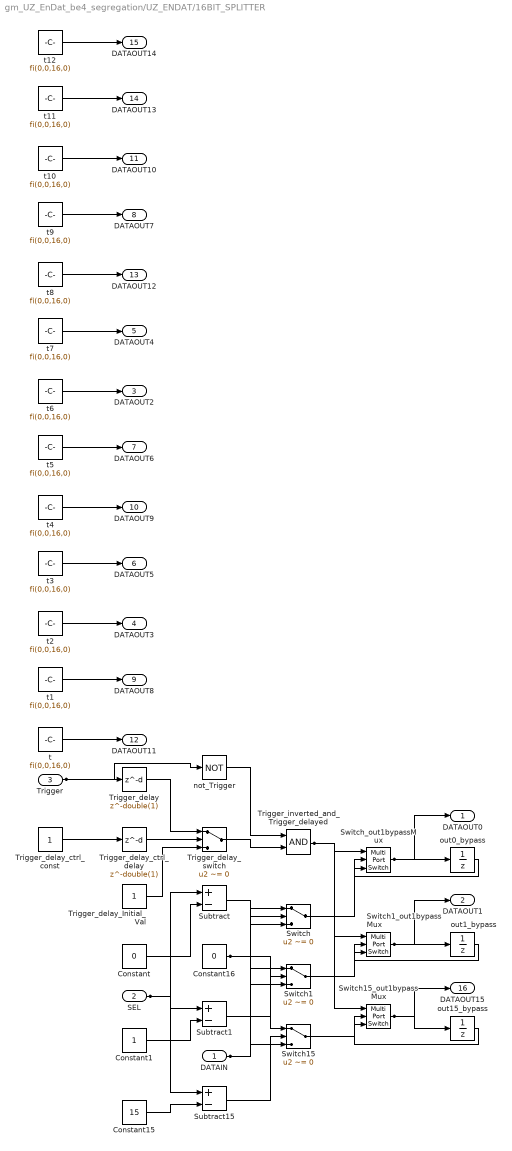
== system gm_UZ_EnDat_be4_segregation/UZ_ENDAT/16BIT_SPLITTER ==
  DATAIN : Inport  OutDataTypeStr=uint16  PortDimensions=1  SampleTime=1e-08
  SEL : Inport  Port=2  OutDataTypeStr=fixdt(0, 4, 0)  PortDimensions=1  SampleTime=1e-08
  Trigger : Inport  Port=3  OutDataTypeStr=boolean  SampleTime=1e-08
  Constant : Constant  Value=0  OutDataTypeStr=fixdt(0, 4, 0)  SampleTime=1e-08
  Constant1 : Constant  OutDataTypeStr=fixdt(0, 4, 0)  SampleTime=1e-08
  Constant15 : Constant  Value=15  OutDataTypeStr=fixdt(0, 4, 0)  SampleTime=1e-08
  Constant16 : Constant  Value=0  OutDataTypeStr=uint16  SampleTime=1e-08
  Subtract : Sum  Inputs=+-  OutDataTypeStr=fixdt(0, 4, 0)  AccumDataTypeStr=fixdt(1, 5, 0)  SampleTime=1e-08
  Subtract1 : Sum  Inputs=+-  OutDataTypeStr=fixdt(0, 4, 0)  AccumDataTypeStr=fixdt(1, 5, 0)  SampleTime=1e-08
  Subtract15 : Sum  Inputs=+-  OutDataTypeStr=fixdt(0, 4, 0)  AccumDataTypeStr=fixdt(1, 5, 0)  SampleTime=1e-08
  Switch : Switch  Criteria=u2 ~= 0  Threshold=double(0)  OutDataTypeStr=uint16  SampleTime=1e-08  SaturateOnIntegerOverflow=off  InputSameDT=off
  Switch1 : Switch  Criteria=u2 ~= 0  Threshold=double(0)  OutDataTypeStr=uint16  SampleTime=1e-08  SaturateOnIntegerOverflow=off  InputSameDT=off
  Switch15 : Switch  Criteria=u2 ~= 0  Threshold=double(0)  OutDataTypeStr=uint16  SampleTime=1e-08  SaturateOnIntegerOverflow=off  InputSameDT=off
  Switch15_out1bypassMux : MultiPortSwitch  DataPortOrder=Zero-based contiguous  Inputs=2  zeroidx=on  OutDataTypeStr=uint16  SampleTime=1e-08  SaturateOnIntegerOverflow=off  InputSameDT=off
  Switch1_out1bypassMux : MultiPortSwitch  DataPortOrder=Zero-based contiguous  Inputs=2  zeroidx=on  OutDataTypeStr=uint16  SampleTime=1e-08  SaturateOnIntegerOverflow=off  InputSameDT=off
  Switch_out1bypassMux : MultiPortSwitch  DataPortOrder=Zero-based contiguous  Inputs=2  zeroidx=on  OutDataTypeStr=uint16  SampleTime=1e-08  SaturateOnIntegerOverflow=off  InputSameDT=off
  Trigger_delay : Delay  DelayLength=double(1)  InitialCondition=0
  Trigger_delay_Initial_Val : Constant  OutDataTypeStr=boolean  SampleTime=1e-08
  Trigger_delay_ctrl_const : Constant  OutDataTypeStr=boolean  SampleTime=1e-08
  Trigger_delay_ctrl_delay : Delay  DelayLength=double(1)  InitialCondition=0
  Trigger_delay_switch : Switch  Criteria=u2 ~= 0  Threshold=double(0)  OutDataTypeStr=boolean  SampleTime=1e-08  SaturateOnIntegerOverflow=off  InputSameDT=off
  Trigger_inverted_and_Trigger_delayed : Logic  AllPortsSameDT=off  OutDataTypeStr=boolean  SampleTime=1e-08
  not_Trigger : Logic  Operator=NOT  Inputs=1  AllPortsSameDT=off  OutDataTypeStr=boolean  SampleTime=1e-08
  out0_bypass : UnitDelay  InitialCondition="fi(0,0,16,0,\"hex\",\"0000\")"  SampleTime=1e-08
  out15_bypass : UnitDelay  InitialCondition="fi(0,0,16,0,\"hex\",\"0000\")"  SampleTime=1e-08
  out1_bypass : UnitDelay  InitialCondition="fi(0,0,16,0,\"hex\",\"0000\")"  SampleTime=1e-08
  t{,1..12} (13 alike) : Constant  Value=fi(0,0,16,0)  OutDataTypeStr=uint16  SampleTime=1e-08
  DATAOUT0 : Outport  SampleTime=1e-08  InitialOutput=0
  DATAOUT1 : Outport  Port=2  SampleTime=1e-08  InitialOutput=0
  DATAOUT2 : Outport  Port=3  SampleTime=1e-08  InitialOutput=0
  DATAOUT3 : Outport  Port=4  SampleTime=1e-08  InitialOutput=0
  DATAOUT4 : Outport  Port=5  SampleTime=1e-08  InitialOutput=0
  DATAOUT5 : Outport  Port=6  SampleTime=1e-08  InitialOutput=0
  DATAOUT6 : Outport  Port=7  SampleTime=1e-08  InitialOutput=0
  DATAOUT7 : Outport  Port=8  SampleTime=1e-08  InitialOutput=0
  DATAOUT8 : Outport  Port=9  SampleTime=1e-08  InitialOutput=0
  DATAOUT9 : Outport  Port=10  SampleTime=1e-08  InitialOutput=0
  DATAOUT10 : Outport  Port=11  SampleTime=1e-08  InitialOutput=0
  DATAOUT11 : Outport  Port=12  SampleTime=1e-08  InitialOutput=0
  DATAOUT12 : Outport  Port=13  SampleTime=1e-08  InitialOutput=0
  DATAOUT13 : Outport  Port=14  SampleTime=1e-08  InitialOutput=0
  DATAOUT14 : Outport  Port=15  SampleTime=1e-08  InitialOutput=0
  DATAOUT15 : Outport  Port=16  SampleTime=1e-08  InitialOutput=0
  wires:
  Trigger/1 -> not_Trigger/1, Trigger_delay/1
  DATAIN/1 -> Switch15/3, Switch1/3, Switch/3
  SEL/1 -> Subtract15/1, Subtract1/1, Subtract/1
  Switch_out1bypassMux/1 -> DATAOUT0/1, out0_bypass/1
  Switch1_out1bypassMux/1 -> DATAOUT1/1, out1_bypass/1
  t6/1 -> DATAOUT2/1
  t2/1 -> DATAOUT3/1
  t7/1 -> DATAOUT4/1
  t3/1 -> DATAOUT5/1
  t5/1 -> DATAOUT6/1
  t9/1 -> DATAOUT7/1
  t1/1 -> DATAOUT8/1
  t4/1 -> DATAOUT9/1
  t10/1 -> DATAOUT10/1
  t/1 -> DATAOUT11/1
  t8/1 -> DATAOUT12/1
  t11/1 -> DATAOUT13/1
  t12/1 -> DATAOUT14/1
  Switch15_out1bypassMux/1 -> DATAOUT15/1, out15_bypass/1
  Trigger_delay_switch/1 -> Trigger_inverted_and_Trigger_delayed/2
  not_Trigger/1 -> Trigger_inverted_and_Trigger_delayed/1
  Trigger_inverted_and_Trigger_delayed/1 -> Switch_out1bypassMux/1, Switch1_out1bypassMux/1, Switch15_out1bypassMux/1
  Trigger_delay/1 -> Trigger_delay_switch/1
  Trigger_delay_Initial_Val/1 -> Trigger_delay_switch/3
  Trigger_delay_ctrl_delay/1 -> Trigger_delay_switch/2
  Subtract/1 -> Switch/2
  Subtract1/1 -> Switch1/2
  Subtract15/1 -> Switch15/2
  Constant/1 -> Subtract/2
  Constant1/1 -> Subtract1/2
  Constant15/1 -> Subtract15/2
  Constant16/1 -> Switch15/1, Switch1/1, Switch/1
  out15_bypass/1 -> Switch15_out1bypassMux/2
  Switch15/1 -> Switch15_out1bypassMux/3
  out0_bypass/1 -> Switch_out1bypassMux/2
  Switch/1 -> Switch_out1bypassMux/3
  out1_bypass/1 -> Switch1_out1bypassMux/2
  Switch1/1 -> Switch1_out1bypassMux/3
  Trigger_delay_ctrl_const/1 -> Trigger_delay_ctrl_delay/1

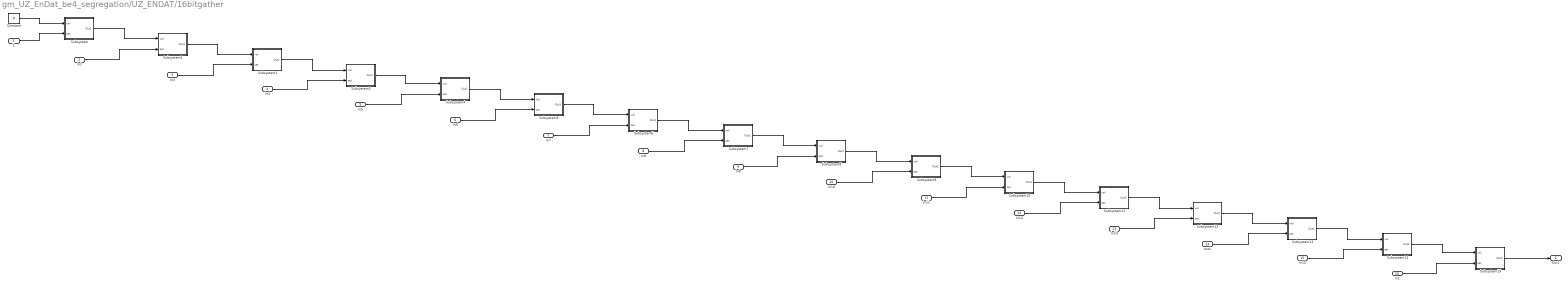
== system gm_UZ_EnDat_be4_segregation/UZ_ENDAT/16bitgather ==
  1 : Inport  OutDataTypeStr=boolean  PortDimensions=1  SampleTime=1e-08
  In2 : Inport  Port=2  OutDataTypeStr=boolean  PortDimensions=1  SampleTime=1e-08
  In3 : Inport  Port=3  OutDataTypeStr=boolean  PortDimensions=1  SampleTime=1e-08
  In4 : Inport  Port=4  OutDataTypeStr=boolean  PortDimensions=1  SampleTime=1e-08
  In5 : Inport  Port=5  OutDataTypeStr=boolean  PortDimensions=1  SampleTime=1e-08
  In6 : Inport  Port=6  OutDataTypeStr=boolean  PortDimensions=1  SampleTime=1e-08
  In7 : Inport  Port=7  OutDataTypeStr=boolean  PortDimensions=1  SampleTime=1e-08
  In8 : Inport  Port=8  OutDataTypeStr=boolean  PortDimensions=1  SampleTime=1e-08
  In9 : Inport  Port=9  OutDataTypeStr=boolean  PortDimensions=1  SampleTime=1e-08
  In10 : Inport  Port=10  OutDataTypeStr=boolean  PortDimensions=1  SampleTime=1e-08
  In11 : Inport  Port=11  OutDataTypeStr=boolean  PortDimensions=1  SampleTime=1e-08
  In12 : Inport  Port=12  OutDataTypeStr=boolean  PortDimensions=1  SampleTime=1e-08
  In13 : Inport  Port=13  OutDataTypeStr=boolean  PortDimensions=1  SampleTime=1e-08
  wrok : Inport  Port=14  OutDataTypeStr=boolean  PortDimensions=1  SampleTime=1e-08
  In15 : Inport  Port=15  OutDataTypeStr=boolean  PortDimensions=1  SampleTime=1e-08
  In1 : Inport  Port=16  OutDataTypeStr=boolean  PortDimensions=1  SampleTime=1e-08
  Constant : Constant  Value=0  OutDataTypeStr=uint16  SampleTime=1e-08
  Subsystem : Subsystem
  Subsystem1 : Subsystem
  Subsystem10 : Subsystem
  Subsystem11 : Subsystem
  Subsystem12 : Subsystem
  Subsystem13 : Subsystem
  Subsystem14 : Subsystem
  Subsystem15 : Subsystem
  Subsystem2 : Subsystem
  Subsystem3 : Subsystem
  Subsystem4 : Subsystem
  Subsystem5 : Subsystem
  Subsystem6 : Subsystem
  Subsystem7 : Subsystem
  Subsystem8 : Subsystem
  Subsystem9 : Subsystem
  Out1 : Outport  SampleTime=1e-08
  wires:
  1/1 -> Subsystem/2(set)
  In2/1 -> Subsystem1/2(set)
  In3/1 -> Subsystem2/2(set)
  In4/1 -> Subsystem3/2(set)
  In5/1 -> Subsystem4/2(set)
  In6/1 -> Subsystem5/2(set)
  In7/1 -> Subsystem6/2(set)
  In8/1 -> Subsystem7/2(set)
  In9/1 -> Subsystem8/2(set)
  In10/1 -> Subsystem9/2(set)
  In11/1 -> Subsystem10/2(set)
  In12/1 -> Subsystem11/2(set)
  In13/1 -> Subsystem12/2(set)
  wrok/1 -> Subsystem13/2(set)
  In15/1 -> Subsystem14/2(set)
  In1/1 -> Subsystem15/2(set)
  Constant/1 -> Subsystem/1(val)
  Subsystem/1(Out1) -> Subsystem1/1(val)
  Subsystem1/1(Out1) -> Subsystem2/1(val)
  Subsystem10/1(Out1) -> Subsystem11/1(val)
  Subsystem11/1(Out1) -> Subsystem12/1(val)
  Subsystem12/1(Out1) -> Subsystem13/1(val)
  Subsystem13/1(Out1) -> Subsystem14/1(val)
  Subsystem14/1(Out1) -> Subsystem15/1(val)
  Subsystem15/1(Out1) -> Out1/1
  Subsystem2/1(Out1) -> Subsystem3/1(val)
  Subsystem3/1(Out1) -> Subsystem4/1(val)
  Subsystem4/1(Out1) -> Subsystem5/1(val)
  Subsystem5/1(Out1) -> Subsystem6/1(val)
  Subsystem6/1(Out1) -> Subsystem7/1(val)
  Subsystem7/1(Out1) -> Subsystem8/1(val)
  Subsystem8/1(Out1) -> Subsystem9/1(val)
  Subsystem9/1(Out1) -> Subsystem10/1(val)

== system gm_UZ_EnDat_be4_segregation/UZ_ENDAT/5timestorage ==
  DATA : Inport  OutDataTypeStr=fixdt(0, 64, 0)  PortDimensions=1  SampleTime=1e-08
  wrok : Inport  Port=2  OutMin=0  OutMax=1  OutDataTypeStr=boolean  PortDimensions=1  SampleTime=1e-08
  Compare To Constant : Subsystem  mask(Compare To Constant){relop===, const=double(0), OutDataTypeStr=boolean, ZeroCross=on}
      mask prompts: relop "Simulink:masks:Operator_MP"; const "Simulink:masks:ConstantValue_MP"; OutDataTypeStr "Simulink:masks:OutputDataType_MP"; ZeroCross "Simulink:masks:EnableZerocrossingDetection_MP"
      mask help: Simulink:masks:CompareToConstant_MD
      mask init:
      | OutDataTypeStr = 'boolean';
      | ZeroCross = 'on';
      | blkName = 'UZ_EnDat_be4_segregation/UZ_ENDAT/5timestorage/Compare\nTo Constant';
      | const = double(0);
      | const_str = '0';
      | const_val = double(0);
      | relop = '==';
      | setValue = 'boolean';
      | str = '== 0';
      mask TypeOptions relop: == | ~= | < | <= | >= | >
      mask TypeOptions OutDataTypeStr: Simulink:masks:uint8 | Simulink:masks:boolean
      mask Callback ZeroCross: sl('zeroCrossEnable', gcbh);
      mask Display: disp(str)
  Compare To Constant1 : Subsystem  mask(Compare To Constant){relop===, const=double(1), OutDataTypeStr=boolean, ZeroCross=on}
      mask prompts: relop "Simulink:masks:Operator_MP"; const "Simulink:masks:ConstantValue_MP"; OutDataTypeStr "Simulink:masks:OutputDataType_MP"; ZeroCross "Simulink:masks:EnableZerocrossingDetection_MP"
      mask help: Simulink:masks:CompareToConstant_MD
      mask init:
      | OutDataTypeStr = 'boolean';
      | ZeroCross = 'on';
      | blkName = 'UZ_EnDat_be4_segregation/UZ_ENDAT/5timestorage/Compare\nTo Constant1';
      | const = double(1);
      | const_str = '1';
      | const_val = double(1);
      | relop = '==';
      | setValue = 'boolean';
      | str = '== 1';
      mask TypeOptions relop: == | ~= | < | <= | >= | >
      mask TypeOptions OutDataTypeStr: Simulink:masks:uint8 | Simulink:masks:boolean
      mask Callback ZeroCross: sl('zeroCrossEnable', gcbh);
      mask Display: disp(str)
  Compare To Constant2 : Subsystem  mask(Compare To Constant){relop===, const=double(2), OutDataTypeStr=boolean, ZeroCross=on}
      mask prompts: relop "Simulink:masks:Operator_MP"; const "Simulink:masks:ConstantValue_MP"; OutDataTypeStr "Simulink:masks:OutputDataType_MP"; ZeroCross "Simulink:masks:EnableZerocrossingDetection_MP"
      mask help: Simulink:masks:CompareToConstant_MD
      mask init:
      | OutDataTypeStr = 'boolean';
      | ZeroCross = 'on';
      | blkName = 'UZ_EnDat_be4_segregation/UZ_ENDAT/5timestorage/Compare\nTo Constant2';
      | const = double(2);
      | const_str = '2';
      | const_val = double(2);
      | relop = '==';
      | setValue = 'boolean';
      | str = '== 2';
      mask TypeOptions relop: == | ~= | < | <= | >= | >
      mask TypeOptions OutDataTypeStr: Simulink:masks:uint8 | Simulink:masks:boolean
      mask Callback ZeroCross: sl('zeroCrossEnable', gcbh);
      mask Display: disp(str)
  Compare To Constant3 : Subsystem  mask(Compare To Constant){relop===, const=double(3), OutDataTypeStr=boolean, ZeroCross=on}
      mask prompts: relop "Simulink:masks:Operator_MP"; const "Simulink:masks:ConstantValue_MP"; OutDataTypeStr "Simulink:masks:OutputDataType_MP"; ZeroCross "Simulink:masks:EnableZerocrossingDetection_MP"
      mask help: Simulink:masks:CompareToConstant_MD
      mask init:
      | OutDataTypeStr = 'boolean';
      | ZeroCross = 'on';
      | blkName = 'UZ_EnDat_be4_segregation/UZ_ENDAT/5timestorage/Compare\nTo Constant3';
      | const = double(3);
      | const_str = '3';
      | const_val = double(3);
      | relop = '==';
      | setValue = 'boolean';
      | str = '== 3';
      mask TypeOptions relop: == | ~= | < | <= | >= | >
      mask TypeOptions OutDataTypeStr: Simulink:masks:uint8 | Simulink:masks:boolean
      mask Callback ZeroCross: sl('zeroCrossEnable', gcbh);
      mask Display: disp(str)
  Compare To Constant4 : Subsystem  mask(Compare To Constant){relop===, const=double(4), OutDataTypeStr=boolean, ZeroCross=on}
      mask prompts: relop "Simulink:masks:Operator_MP"; const "Simulink:masks:ConstantValue_MP"; OutDataTypeStr "Simulink:masks:OutputDataType_MP"; ZeroCross "Simulink:masks:EnableZerocrossingDetection_MP"
      mask help: Simulink:masks:CompareToConstant_MD
      mask init:
      | OutDataTypeStr = 'boolean';
      | ZeroCross = 'on';
      | blkName = 'UZ_EnDat_be4_segregation/UZ_ENDAT/5timestorage/Compare\nTo Constant4';
      | const = double(4);
      | const_str = '4';
      | const_val = double(4);
      | relop = '==';
      | setValue = 'boolean';
      | str = '== 4';
      mask TypeOptions relop: == | ~= | < | <= | >= | >
      mask TypeOptions OutDataTypeStr: Simulink:masks:uint8 | Simulink:masks:boolean
      mask Callback ZeroCross: sl('zeroCrossEnable', gcbh);
      mask Display: disp(str)
  Multiport Switch : MultiPortSwitch  DataPortOrder=Zero-based contiguous  Inputs=5  DiagnosticForDefault=None  zeroidx=on  OutDataTypeStr=fixdt(0, 64, 0)  SampleTime=1e-08  SaturateOnIntegerOverflow=off  InputSameDT=off
  Storage20 : Subsystem
  Storage20_term1 : Terminator
  Storage21 : Subsystem
  Storage21_term1 : Terminator
  Storage22 : Subsystem
  Storage22_term1 : Terminator
  Storage23 : Subsystem
  Storage23_term1 : Terminator
  Storage24 : Subsystem
  Storage24_term1 : Terminator
  Triggered Subsystem : Subsystem
  t{,1..3} (4 alike) : Constant  Value=fi(0,0,64,0)  OutDataTypeStr=fixdt(0, 64, 0)  SampleTime=1e-08
  t0 : Outport  SampleTime=1e-08
  t-1 : Outport  Port=2  SampleTime=1e-08
  t-2 : Outport  Port=3  SampleTime=1e-08
  t-3 : Outport  Port=4  SampleTime=1e-08
  t-4 : Outport  Port=5  SampleTime=1e-08
  wires:
  DATA/1 -> Storage24/1(Data), Storage23/1(Data), Storage22/1(Data), Storage21/1(Data), Storage20/1(Data)
  wrok/1 -> Triggered Subsystem/1(Trigger)
  Compare To Constant/1(y) -> Storage20/2(Write)
  Compare To Constant1/1(y) -> Storage21/2(Write)
  Compare To Constant2/1(y) -> Storage22/2(Write)
  Compare To Constant3/1(y) -> Storage23/2(Write)
  Compare To Constant4/1(y) -> Storage24/2(Write)
  Multiport Switch/1 -> t0/1
  t/1 -> t-1/1
  t1/1 -> t-2/1
  t2/1 -> t-3/1
  t3/1 -> t-4/1
  Storage20/1(out) -> Multiport Switch/2
  Storage21/1(out) -> Multiport Switch/3
  Storage22/1(out) -> Multiport Switch/4
  Storage23/1(out) -> Multiport Switch/5
  Storage24/1(out) -> Multiport Switch/6
  Triggered Subsystem/1(Out1) -> Multiport Switch/1, Compare To Constant4/1(u), Compare To Constant3/1(u), Compare To Constant2/1(u), Compare To Constant1/1(u), Compare To Constant/1(u)
  Storage20/2(wrok) -> Storage20_term1/1
  Storage21/2(wrok) -> Storage21_term1/1
  Storage22/2(wrok) -> Storage22_term1/1
  Storage23/2(wrok) -> Storage23_term1/1
  Storage24/2(wrok) -> Storage24_term1/1

== system gm_UZ_EnDat_be4_segregation/UZ_ENDAT/CLKCNTER_ACT ==
  CLK : Inport  OutDataTypeStr=boolean  PortDimensions=1  SampleTime=1e-08
  CLK2CNT : Inport  Port=2  OutDataTypeStr=boolean  PortDimensions=1  SampleTime=1e-08
  ResetCNT : Inport  Port=3  OutDataTypeStr=boolean  PortDimensions=1  SampleTime=1e-08
  Delay1 : Delay  DelayLength=double(1)  InitialCondition=0  SampleTime=1e-08
  Delay1_enbsw : Switch  Criteria=u2 ~= 0  Threshold=double(0)  OutDataTypeStr=uint32  SampleTime=1e-08  SaturateOnIntegerOverflow=off  InputSameDT=off
  Positional_Counter : Subsystem
  SetZero32 : Subsystem
  delayMatch : Delay  DelayLength=double(2)  InitialCondition=0  SampleTime=1e-08
  stateControl : Constant  OutDataTypeStr=boolean  SampleTime=1e-08
  CNT : Outport  SampleTime=1e-08
  wires:
  stateControl/1 -> delayMatch/1
  ResetCNT/1 -> SetZero32/2(setzero)
  CLK/1 -> SetZero32/3(Trigger)
  Positional_Counter/1(divider) -> SetZero32/1(valin)
  delayMatch/1 -> Delay1_enbsw/2
  CLK2CNT/1 -> Positional_Counter/2(Trigger)
  Delay1/1 -> Delay1_enbsw/3, Positional_Counter/1(valueout), CNT/1
  SetZero32/1(valueout) -> Delay1_enbsw/1
  Delay1_enbsw/1 -> Delay1/1

== system gm_UZ_EnDat_be4_segregation/UZ_ENDAT/CLKCNTER_RAMPUP ==
  CLK : Inport  OutDataTypeStr=boolean  PortDimensions=1  SampleTime=1e-08
  CLK2CNT : Inport  Port=2  OutDataTypeStr=boolean  PortDimensions=1  SampleTime=1e-08
  ResetCNT : Inport  Port=3  OutDataTypeStr=boolean  PortDimensions=1  SampleTime=1e-08
  Delay1 : Delay  DelayLength=double(1)  InitialCondition=0  SampleTime=1e-08
  Positional_Counter : Subsystem
  SetZero32 : Subsystem
  CNT : Outport  SampleTime=1e-08
  wires:
  Delay1/1 -> CNT/1, Positional_Counter/1(valueout)
  SetZero32/1(valueout) -> Delay1/1
  CLK2CNT/1 -> Positional_Counter/2(Trigger)
  ResetCNT/1 -> SetZero32/2(setzero)
  CLK/1 -> SetZero32/3(Trigger)
  Positional_Counter/1(divider) -> SetZero32/1(valin)

== system gm_UZ_EnDat_be4_segregation/UZ_ENDAT/CLKDIV1 ==
  CLK1 : Inport  OutDataTypeStr=boolean  PortDimensions=1  SampleTime=1e-08
  Delay : Delay  DelayLength=double(1)  InitialCondition=0  SampleTime=1e-08
  Logical Operator1 : Logic  Operator=NOT  Inputs=1  AllPortsSameDT=off  OutDataTypeStr=boolean  SampleTime=1e-08
  Triggered Subsystem : Subsystem
  CLK/2 : Outport  OutDataTypeStr=boolean  SampleTime=1e-08  VectorParamsAs1DForOutWhenUnconnected=off
  wires:
  Logical Operator1/1 -> CLK/2/1, Delay/1
  Triggered Subsystem/1(Q) -> Logical Operator1/1
  CLK1/1 -> Triggered Subsystem/2(Trigger)
  Delay/1 -> Triggered Subsystem/1(D)

== system gm_UZ_EnDat_be4_segregation/UZ_ENDAT/CLKDIV2 ==
  CLK1 : Inport  OutDataTypeStr=boolean  PortDimensions=1  SampleTime=1e-08
  CLK/2 : Outport  OutDataTypeStr=boolean  SampleTime=1e-08  VectorParamsAs1DForOutWhenUnconnected=off
  wires:
  CLK1/1 -> CLK/2/1

== system gm_UZ_EnDat_be4_segregation/UZ_ENDAT/CLKDIV3 ==
  CLK1 : Inport  OutDataTypeStr=boolean  PortDimensions=1  SampleTime=1e-08
  Delay : Delay  DelayLength=double(1)  InitialCondition=0  SampleTime=1e-08
  Logical Operator1 : Logic  Operator=NOT  Inputs=1  AllPortsSameDT=off  OutDataTypeStr=boolean  SampleTime=1e-08
  Triggered Subsystem : Subsystem
  CLK/2 : Outport  OutDataTypeStr=boolean  SampleTime=1e-08  VectorParamsAs1DForOutWhenUnconnected=off
  wires:
  Logical Operator1/1 -> CLK/2/1, Delay/1
  Triggered Subsystem/1(Q) -> Logical Operator1/1
  CLK1/1 -> Triggered Subsystem/2(Trigger)
  Delay/1 -> Triggered Subsystem/1(D)

== system gm_UZ_EnDat_be4_segregation/UZ_ENDAT/CLKDIV4 ==
  CLK1 : Inport  OutDataTypeStr=boolean  PortDimensions=1  SampleTime=1e-08
  Delay : Delay  DelayLength=double(1)  InitialCondition=0  SampleTime=1e-08
  Logical Operator1 : Logic  Operator=NOT  Inputs=1  AllPortsSameDT=off  OutDataTypeStr=boolean  SampleTime=1e-08
  Triggered Subsystem : Subsystem
  CLK/2 : Outport  OutDataTypeStr=boolean  SampleTime=1e-08  VectorParamsAs1DForOutWhenUnconnected=off
  wires:
  Logical Operator1/1 -> CLK/2/1, Delay/1
  Triggered Subsystem/1(Q) -> Logical Operator1/1
  CLK1/1 -> Triggered Subsystem/2(Trigger)
  Delay/1 -> Triggered Subsystem/1(D)

== system gm_UZ_EnDat_be4_segregation/UZ_ENDAT/CLKDIV5 ==
  CLK1 : Inport  OutDataTypeStr=boolean  PortDimensions=1  SampleTime=1e-08
  Delay : Delay  DelayLength=double(1)  InitialCondition=0  SampleTime=1e-08
  Logical Operator1 : Logic  Operator=NOT  Inputs=1  AllPortsSameDT=off  OutDataTypeStr=boolean  SampleTime=1e-08
  Triggered Subsystem : Subsystem
  CLK/2 : Outport  OutDataTypeStr=boolean  SampleTime=1e-08  VectorParamsAs1DForOutWhenUnconnected=off
  wires:
  Logical Operator1/1 -> CLK/2/1, Delay/1
  Triggered Subsystem/1(Q) -> Logical Operator1/1
  CLK1/1 -> Triggered Subsystem/2(Trigger)
  Delay/1 -> Triggered Subsystem/1(D)

== system gm_UZ_EnDat_be4_segregation/UZ_ENDAT/CLKDIV6 ==
  CLK1 : Inport  OutDataTypeStr=boolean  PortDimensions=1  SampleTime=1e-08
  Delay : Delay  DelayLength=double(1)  InitialCondition=0  SampleTime=1e-08
  Logical Operator1 : Logic  Operator=NOT  Inputs=1  AllPortsSameDT=off  OutDataTypeStr=boolean  SampleTime=1e-08
  Triggered Subsystem : Subsystem
  CLK/2 : Outport  OutDataTypeStr=boolean  SampleTime=1e-08  VectorParamsAs1DForOutWhenUnconnected=off
  wires:
  Logical Operator1/1 -> CLK/2/1, Delay/1
  Triggered Subsystem/1(Q) -> Logical Operator1/1
  CLK1/1 -> Triggered Subsystem/2(Trigger)
  Delay/1 -> Triggered Subsystem/1(D)
